simulink model "que4"  (R2020b)
settings: Solver=VariableStepAuto  StartTime=0.0  StopTime=10.0  RelTol=1e-3
settings Model: Creator=hp  LastModifiedBy=hp

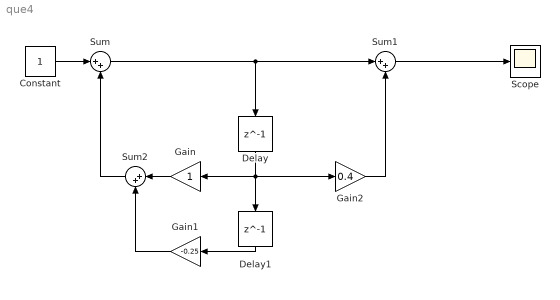
== system que4 ==
  Constant : Constant
  Delay : Delay  DelayLength=1  InitialCondition=0
  Delay1 : Delay  DelayLength=1  InitialCondition=0
  Gain : Gain
  Gain1 : Gain  Gain=-0.25
  Gain2 : Gain  Gain=0.4
  Scope : Scope
  Sum : Sum  Inputs=|++
  Sum1 : Sum  Inputs=|++
  Sum2 : Sum  Inputs=|++
  wires:
  Sum2/1 -> Sum/2
  Sum/1 -> Delay/1, Sum1/1
  Delay/1 -> Gain2/1, Delay1/1, Gain/1
  Gain/1 -> Sum2/1
  Delay1/1 -> Gain1/1
  Gain1/1 -> Sum2/2
  Gain2/1 -> Sum1/2
  Sum1/1 -> Scope/1
  Constant/1 -> Sum/1
